simulink model "pmsm_dynamic"  (R2016a)
settings: Solver=ode45  StartTime=0.0  StopTime=2  MaxStep=1e-3  RelTol=1e-3
undefined symbols (not defined in the file): Kp, L, lambda_m, P, r, Tmref, Vdc, wz
libraries: simulink x2
settings Model: Creator=Gorkem  LastModifiedBy=Gorkem
settings GRTTargetCC: GeneratePreprocessorConditionals=Use local settings

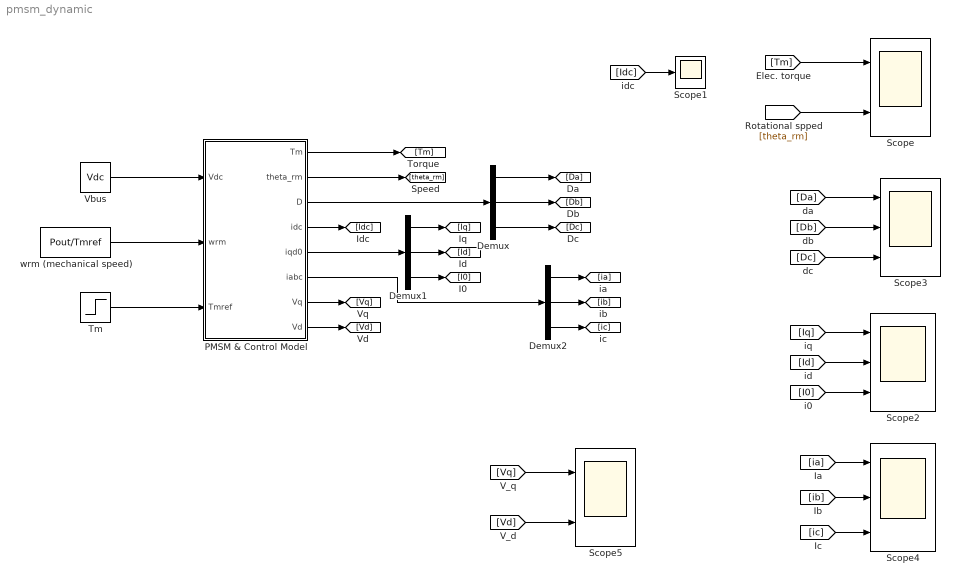
== system pmsm_dynamic ==
  Demux : Demux  Outputs=3
  Demux1 : Demux  Outputs=3
  Demux2 : Demux  Outputs=3
  PMSM & Control Model : Subsystem
  Scope : Scope  NumInputPorts=2
  Scope1 : Scope
  Scope2 : Scope  NumInputPorts=3
  Scope3 : Scope  NumInputPorts=3
  Scope4 : Scope  NumInputPorts=3
  Scope5 : Scope  NumInputPorts=2
  Tm : Step  Time=0.4  After=Tmref  SampleTime=0
  Vbus : Constant  Value=Vdc
  wrm (mechanical speed) : Constant  Value=Pout/Tmref
  wires:
  wrm (mechanical speed)/1 -> PMSM & Control Model/2(wrm)
  Vbus/1 -> PMSM & Control Model/1(Vdc)
  Tm/1 -> PMSM & Control Model/3(Tmref)
  PMSM & Control Model/3(D) -> Demux/1
  PMSM & Control Model/5(iqd0) -> Demux1/1
  PMSM & Control Model/6(iabc) -> Demux2/1
  PMSM & Control Model/2(theta_rm) -> [theta_rm]
  PMSM & Control Model/1(Tm) -> [Tm]
  Demux/3 -> [Dc]
  Demux/2 -> [Db]
  Demux/1 -> [Da]
  Demux1/1 -> [Iq]
  Demux1/2 -> [Id]
  Demux1/3 -> [I0]
  PMSM & Control Model/7(Vq) -> [Vq]
  PMSM & Control Model/8(Vd) -> [Vd]
  Demux2/2 -> [ib]
  Demux2/1 -> [ia]
  Demux2/3 -> [ic]
  PMSM & Control Model/4(idc) -> [Idc]
  [Tm] -> Scope/1
  [theta_rm] -> Scope/2
  [Da] -> Scope3/1
  [Db] -> Scope3/2
  [Dc] -> Scope3/3
  [Iq] -> Scope2/1
  [Id] -> Scope2/2
  [I0] -> Scope2/3
  [Idc] -> Scope1/1
  [ia] -> Scope4/1
  [ib] -> Scope4/2
  [ic] -> Scope4/3
  [Vq] -> Scope5/1
  [Vd] -> Scope5/2

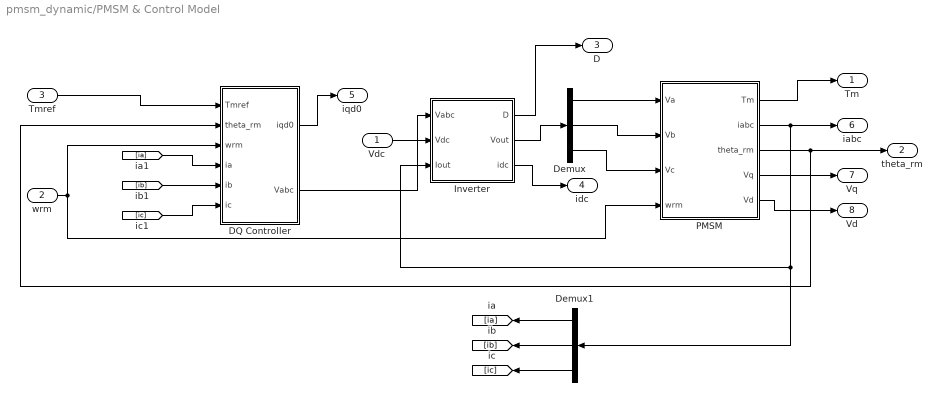
== system pmsm_dynamic/PMSM & Control Model ==
  Vdc : Inport
  wrm : Inport  Port=2
  Tmref : Inport  Port=3
  DQ Controller : Subsystem
  Demux : Demux  Outputs=3
  Demux1 : Demux  Outputs=3
  Inverter : Subsystem
  PMSM : Subsystem
  Tm : Outport
  theta_rm : Outport  Port=2
  D : Outport  Port=3
  idc : Outport  Port=4
  iqd0 : Outport  Port=5
  iabc : Outport  Port=6
  Vq : Outport  Port=7
  Vd : Outport  Port=8
  wires:
  Vdc/1 -> Inverter/2(Vdc)
  DQ Controller/2(Vabc) -> Inverter/1(Vabc)
  Inverter/1(D) -> D/1
  Demux/3 -> PMSM/3(Vc)
  PMSM/3(theta_rm) -> DQ Controller/2(theta_rm), theta_rm/1
  Inverter/3(idc) -> idc/1
  Tmref/1 -> DQ Controller/1(Tmref)
  wrm/1 -> PMSM/4(wrm), DQ Controller/3(wrm)
  DQ Controller/1(iqd0) -> iqd0/1
  Demux/2 -> PMSM/2(Vb)
  Inverter/2(Vout) -> Demux/1
  PMSM/1(Tm) -> Tm/1
  Demux/1 -> PMSM/1(Va)
  PMSM/4(Vq) -> Vq/1
  PMSM/5(Vd) -> Vd/1
  PMSM/2("iabc ") -> Demux1/1, Inverter/3("Iout "), iabc/1
  Demux1/1 -> [ia]
  Demux1/2 -> [ib]
  Demux1/3 -> [ic]
  [ia] -> DQ Controller/4(ia)
  [ib] -> DQ Controller/5(ib)
  [ic] -> DQ Controller/6(ic)

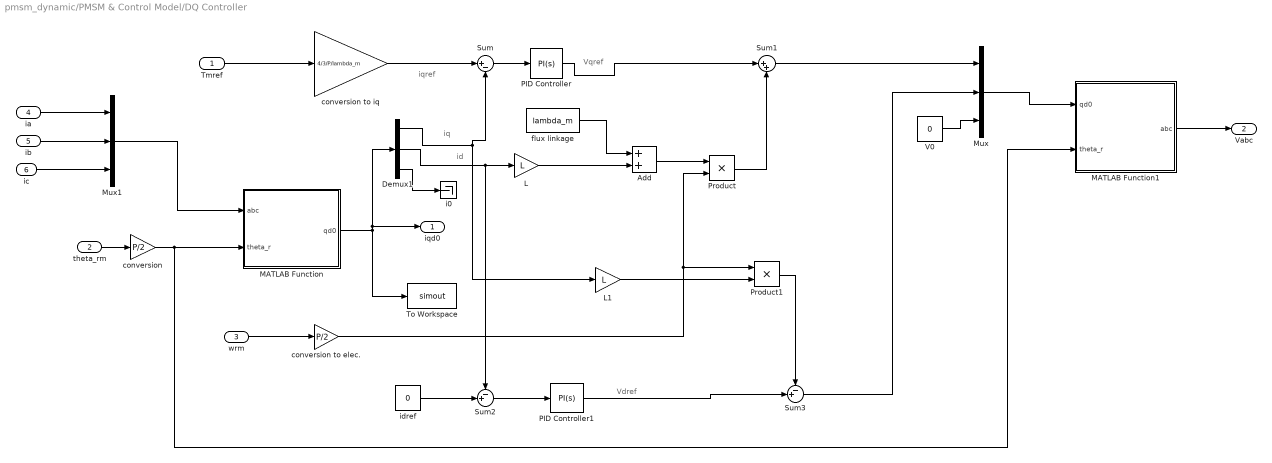
== system pmsm_dynamic/PMSM & Control Model/DQ Controller ==
  note: iqref
  note: Vdref
  note: id
  note: Vqref
  note: iq
  Tmref : Inport
  theta_rm : Inport  Port=2
  wrm : Inport  Port=3
  ia : Inport  Port=4
  ib : Inport  Port=5
  ic : Inport  Port=6
  Add : Sum
  Demux1 : Demux  Outputs=[1 1 1]
  L : Gain  Gain=L
  L1 : Gain  Gain=L
  MATLAB Function : MATLAB Function  TreatAsAtomicUnit=on
  MATLAB Function1 : MATLAB Function  TreatAsAtomicUnit=on
  Mux : Mux  Inputs=[1 1 1]
  Mux1 : Mux  Inputs=[1 1 1]
  PID Controller : simulink/Continuous/PID Controller  Controller=PI  TimeDomain=Continuous-time  SampleTime=-1  IntegratorMethod=Forward Euler  FilterMethod=Forward Euler  Form=Parallel  UseFilter=on  ControllerParametersSource=internal  P=Kp  I=Kp*wz  D=0  N=100  InitialConditionSource=internal  InitialConditionForIntegrator=0  InitialConditionForFilter=0  ExternalReset=none  LimitOutput=off  UpperSaturationLimit=inf  LowerSaturationLimit=-inf  LinearizeAsGain=on  AntiWindupMode=none  Kb=1  TrackingMode=off  Kt=1  PParamMin=[]  PParamMax=[]  IParamMin=[]  IParamMax=[]  DParamMin=[]  DParamMax=[]  NParamMin=[]  NParamMax=[]  KbParamMin=[]  KbParamMax=[]  KtParamMin=[]  KtParamMax=[]  POutMin=[]  POutMax=[]  IOutMin=[]  IOutMax=[]  DOutMin=[]  DOutMax=[]  NOutMin=[]  NOutMax=[]  KbOutMin=[]  KbOutMax=[]  KtOutMin=[]  KtOutMax=[]  IntegratorOutMin=[]  IntegratorOutMax=[]  FilterOutMin=[]  FilterOutMax=[]  SumOutMin=[]  SumOutMax=[]  SumI1OutMin=[]  SumI1OutMax=[]  SumI2OutMin=[]  SumI2OutMax=[]  SumI3OutMin=[]  SumI3OutMax=[]  SumDOutMin=[]  SumDOutMax=[]  SaturationOutMin=[]  SaturationOutMax=[]  IntegratorContinuousStateAttributes=''  IntegratorStateMustResolveToSignalObject=off  IntegratorRTWStateStorageClass=Auto  FilterContinuousStateAttributes=''  FilterStateMustResolveToSignalObject=off  FilterRTWStateStorageClass=Auto  DifferentiatorICPrevScaledInput=0  DifferentiatorOutMin=[]  DifferentiatorOutMax=[]
  PID Controller1 : simulink/Continuous/PID Controller  Controller=PI  TimeDomain=Continuous-time  SampleTime=-1  IntegratorMethod=Forward Euler  FilterMethod=Forward Euler  Form=Parallel  UseFilter=on  ControllerParametersSource=internal  P=Kp  I=Kp*wz  D=0  N=100  InitialConditionSource=internal  InitialConditionForIntegrator=0  InitialConditionForFilter=0  ExternalReset=none  LimitOutput=off  UpperSaturationLimit=inf  LowerSaturationLimit=-inf  LinearizeAsGain=on  AntiWindupMode=none  Kb=1  TrackingMode=off  Kt=1  PParamMin=[]  PParamMax=[]  IParamMin=[]  IParamMax=[]  DParamMin=[]  DParamMax=[]  NParamMin=[]  NParamMax=[]  KbParamMin=[]  KbParamMax=[]  KtParamMin=[]  KtParamMax=[]  POutMin=[]  POutMax=[]  IOutMin=[]  IOutMax=[]  DOutMin=[]  DOutMax=[]  NOutMin=[]  NOutMax=[]  KbOutMin=[]  KbOutMax=[]  KtOutMin=[]  KtOutMax=[]  IntegratorOutMin=[]  IntegratorOutMax=[]  FilterOutMin=[]  FilterOutMax=[]  SumOutMin=[]  SumOutMax=[]  SumI1OutMin=[]  SumI1OutMax=[]  SumI2OutMin=[]  SumI2OutMax=[]  SumI3OutMin=[]  SumI3OutMax=[]  SumDOutMin=[]  SumDOutMax=[]  SaturationOutMin=[]  SaturationOutMax=[]  IntegratorContinuousStateAttributes=''  IntegratorStateMustResolveToSignalObject=off  IntegratorRTWStateStorageClass=Auto  FilterContinuousStateAttributes=''  FilterStateMustResolveToSignalObject=off  FilterRTWStateStorageClass=Auto  DifferentiatorICPrevScaledInput=0  DifferentiatorOutMin=[]  DifferentiatorOutMax=[]
  Product : Product
  Product1 : Product
  Sum : Sum  Inputs=|+-
  Sum1 : Sum  Inputs=|++
  Sum2 : Sum  Inputs=-+|
  Sum3 : Sum  Inputs=-+|
  To Workspace : ToWorkspace  VariableName=simout  SaveFormat=Structure  SampleTime=-1
  V0 : Constant  Value=0
  "conversion " : Gain  Gain=P/2
  conversion to elec. : Gain  Gain=P/2
  conversion to iq : Gain  Gain=4/3/P/lambda_m
  flux linkage : Constant  Value=lambda_m
  i0 : Terminator
  idref : Constant  Value=0
  iqd0 : Outport
  Vabc : Outport  Port=2
  wires:
  wrm/1 -> conversion to elec./1
  theta_rm/1 -> "conversion "/1
  Tmref/1 -> conversion to iq/1
  MATLAB Function/1(qd0) -> Demux1/1, iqd0/1, To Workspace/1
  conversion to iq/1 -> Sum/1
  Demux1/1 -> Sum/2, L1/1
  Sum/1 -> PID Controller/1
  PID Controller/1 -> Sum1/1
  Demux1/2 -> Sum2/1, L/1
  L/1 -> Add/2
  flux linkage/1 -> Add/1
  Add/1 -> Product/1
  conversion to elec./1 -> Product/2, Product1/1
  Product/1 -> Sum1/2
  idref/1 -> Sum2/2
  Sum2/1 -> PID Controller1/1
  L1/1 -> Product1/2
  PID Controller1/1 -> Sum3/2
  Product1/1 -> Sum3/1
  Sum1/1 -> Mux/1
  V0/1 -> Mux/3
  "conversion "/1 -> MATLAB Function1/2(theta_r), MATLAB Function/2(theta_r)
  Demux1/3 -> i0/1
  Mux1/1 -> MATLAB Function/1(abc)
  Sum3/1 -> Mux/2
  Mux/1 -> MATLAB Function1/1(qd0)
  MATLAB Function1/1(abc) -> Vabc/1
  ia/1 -> Mux1/1
  ib/1 -> Mux1/2
  ic/1 -> Mux1/3

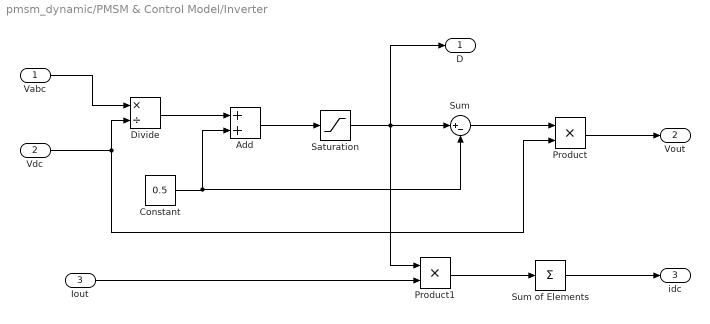
== system pmsm_dynamic/PMSM & Control Model/Inverter ==
  Vabc : Inport
  Vdc : Inport  Port=2
  "Iout " : Inport  Port=3
  Add : Sum
  Constant : Constant  Value=0.5
  Divide : Product  Inputs=*/
  Product : Product
  Product1 : Product
  Saturation : Saturate  UpperLimit=1  LowerLimit=0
  Sum : Sum  Inputs=|+-
  Sum of Elements : Sum  Inputs=+
  D : Outport
  Vout : Outport  Port=2
  idc : Outport  Port=3
  wires:
  Constant/1 -> Sum/2, Add/2
  Vabc/1 -> Divide/1
  Divide/1 -> Add/1
  Product/1 -> Vout/1
  Sum/1 -> Product/1
  "Iout "/1 -> Product1/2
  Product1/1 -> Sum of Elements/1
  Sum of Elements/1 -> idc/1
  Vdc/1 -> Divide/2, Product/2
  Saturation/1 -> D/1, Product1/1, Sum/1
  Add/1 -> Saturation/1

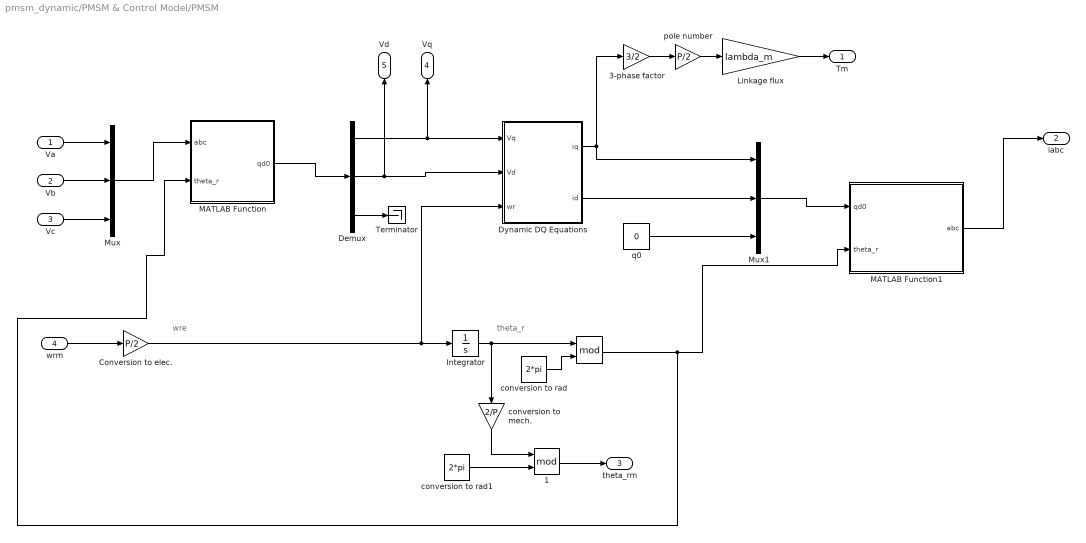
== system pmsm_dynamic/PMSM & Control Model/PMSM ==
  note: theta_r
  note: wre
  Va : Inport
  Vb : Inport  Port=2
  Vc : Inport  Port=3
  wrm : Inport  Port=4
  "  " : Math  Operator=mod  SaturateOnIntegerOverflow=on
  "  1" : Math  Operator=mod  SaturateOnIntegerOverflow=on
  3-phase factor : Gain  Gain=3/2
  Conversion to elec. : Gain  Gain=P/2
  Demux : Demux  Outputs=3
  Dynamic DQ Equations : Subsystem
  Integrator : Integrator
  Linkage flux : Gain  Gain=lambda_m
  MATLAB Function : MATLAB Function  TreatAsAtomicUnit=on
  MATLAB Function1 : MATLAB Function  TreatAsAtomicUnit=on
  Mux : Mux  Inputs=3
  Mux1 : Mux  Inputs=3
  Terminator : Terminator
  conversion to mech. : Gain  Gain=2/P
  conversion to rad : Constant  Value=2*pi
  conversion to rad1 : Constant  Value=2*pi
  pole number : Gain  Gain=P/2
  q0 : Constant  Value=0
  Tm : Outport
  "iabc " : Outport  Port=2
  theta_rm : Outport  Port=3
  Vq : Outport  Port=4
  Vd : Outport  Port=5
  wires:
  "  1"/1 -> theta_rm/1
  "  "/1 -> MATLAB Function/2(theta_r), MATLAB Function1/2(theta_r)
  conversion to mech./1 -> "  1"/1
  conversion to rad1/1 -> "  1"/2
  Integrator/1 -> "  "/1, conversion to mech./1
  MATLAB Function1/1(abc) -> "iabc "/1
  Vc/1 -> Mux/3
  Demux/1 -> Vq/1, Dynamic DQ Equations/1(Vq)
  Va/1 -> Mux/1
  q0/1 -> Mux1/3
  pole number/1 -> Linkage flux/1
  Dynamic DQ Equations/2(id) -> Mux1/2
  conversion to rad/1 -> "  "/2
  Demux/3 -> Terminator/1
  Vb/1 -> Mux/2
  Demux/2 -> Vd/1, Dynamic DQ Equations/2(Vd)
  Dynamic DQ Equations/1(iq) -> Mux1/1, 3-phase factor/1
  Conversion to elec./1 -> Dynamic DQ Equations/3(wr), Integrator/1
  wrm/1 -> Conversion to elec./1
  3-phase factor/1 -> pole number/1
  Linkage flux/1 -> Tm/1
  MATLAB Function/1(qd0) -> Demux/1
  Mux/1 -> MATLAB Function/1(abc)
  Mux1/1 -> MATLAB Function1/1(qd0)

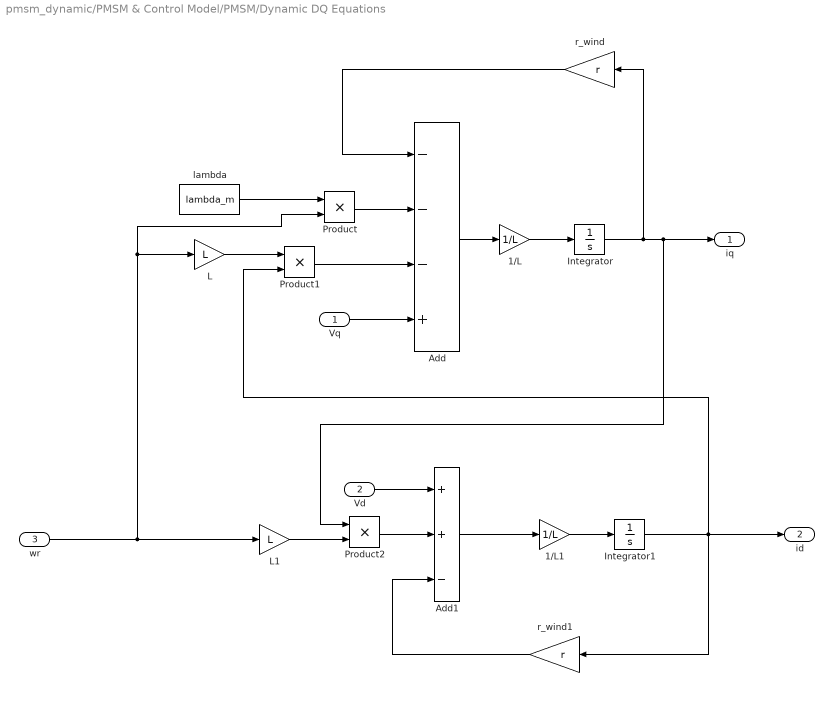
== system pmsm_dynamic/PMSM & Control Model/PMSM/Dynamic DQ Equations ==
  Vq : Inport
  Vd : Inport  Port=2
  wr : Inport  Port=3
  1/L : Gain  Gain=1/L
  1/L1 : Gain  Gain=1/L
  Add : Sum  Inputs=---+
  Add1 : Sum  Inputs=++-
  Integrator : Integrator
  Integrator1 : Integrator
  L : Gain  Gain=L
  L1 : Gain  Gain=L
  Product : Product
  Product1 : Product
  Product2 : Product
  lambda : Constant  Value=lambda_m
  r_wind : Gain  Gain=r
  r_wind1 : Gain  Gain=r
  iq : Outport
  id : Outport  Port=2
  wires:
  1/L/1 -> Integrator/1
  Vq/1 -> Add/4
  r_wind/1 -> Add/1
  Integrator1/1 -> id/1, r_wind1/1, Product1/2
  Vd/1 -> Add1/1
  r_wind1/1 -> Add1/3
  Product1/1 -> Add/3
  Add/1 -> 1/L/1
  Product2/1 -> Add1/2
  L1/1 -> Product2/2
  lambda/1 -> Product/1
  L/1 -> Product1/1
  Product/1 -> Add/2
  wr/1 -> L1/1, L/1, Product/2
  1/L1/1 -> Integrator1/1
  Add1/1 -> 1/L1/1
  Integrator/1 -> r_wind/1, iq/1, Product2/1

== matlab function pmsm_dynamic/PMSM & Control Model/DQ Controller/MATLAB Function1 ==
  data: qd0 input; abc output; theta_r input
function abc = Inverse_DQTransform(qd0, theta_r)
%#codegen

Kr = 2/3*[  cos(theta_r)      cos(theta_r-2*pi/3)     cos(theta_r + 2*pi/3);
            sin(theta_r)      sin(theta_r-2*pi/3)     sin(theta_r + 2*pi/3);
            1/2               1/2                     1/2];
  
abc = Kr\qd0;

== matlab function pmsm_dynamic/PMSM & Control Model/DQ Controller/MATLAB Function ==
  data: abc input; qd0 output; theta_r input
function qd0 = DQTransform(abc, theta_r)
%#codegen

Kr = 2/3*[  cos(theta_r)      cos(theta_r-2*pi/3)     cos(theta_r + 2*pi/3);
            sin(theta_r)      sin(theta_r-2*pi/3)     sin(theta_r + 2*pi/3);
            1/2               1/2                     1/2];
  
qd0 = Kr*abc;

== matlab function pmsm_dynamic/PMSM & Control Model/PMSM/MATLAB Function ==
  data: abc input; qd0 output; theta_r input
function qd0 = DQTransform(abc, theta_r)
%#codegen

Kr = 2/3*[  cos(theta_r)      cos(theta_r-2*pi/3)     cos(theta_r + 2*pi/3);
            sin(theta_r)      sin(theta_r-2*pi/3)     sin(theta_r + 2*pi/3);
            1/2               1/2                     1/2];
  
qd0 = Kr*abc;

== matlab function pmsm_dynamic/PMSM & Control Model/PMSM/MATLAB Function1 ==
  data: qd0 input; abc output; theta_r input
function abc = Inverse_DQTransform(qd0, theta_r)
%#codegen

Kr = 2/3*[  cos(theta_r)      cos(theta_r-2*pi/3)     cos(theta_r + 2*pi/3);
            sin(theta_r)      sin(theta_r-2*pi/3)     sin(theta_r + 2*pi/3);
            1/2               1/2                     1/2];
  
abc = Kr\qd0;
